simulink model "narrow_FM"  (R2020b)
settings: Solver=VariableStepAuto  StartTime=0.0  StopTime=10.0  RelTol=1e-3
undefined symbols (not defined in the file or in its folder): DiscIntNeverNeededParam
libraries: audiosources x3, dspvision x3, dspfdesign x2, simulink x1
settings Model: Creator=MinsooKang  LastModifiedBy=MinsooKang

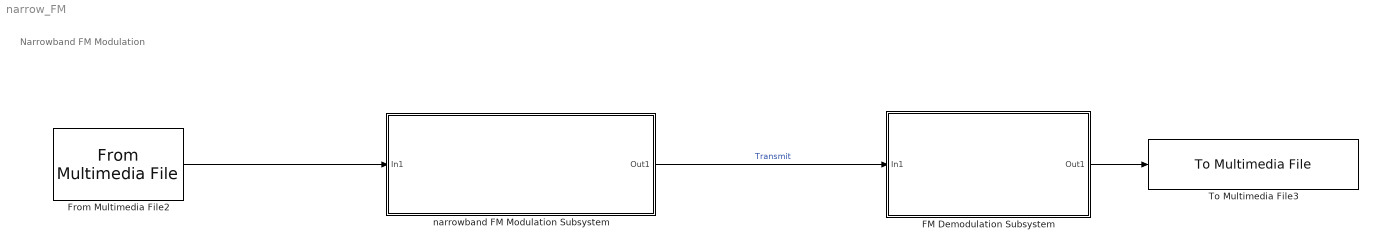
== system narrow_FM ==
  note: Narrowband FM Modulation
  FM Demodulation Subsystem : Subsystem
  From Multimedia File2 : dspvision/From Multimedia File  inputFilename=C:\Users\MinsooKang\Desktop\matlab\audio.flac  readRange=[1 Inf]  loop=on  numPlays=inf  outputStreams=Audio only  videoDataType=single  audioDataType=double  inheritSampleTime=on  userDefinedSampleTime=1/30  noAudioOutput=off  isIntensityVideo=off  fourcc=RGB  colorVideoFormat=Separate color signals  outputEOF=off  dataOrg=Column-major  audioFrameSize=1024  computeAudioFrameSize=off  outSamplingMode=Sample based
  To Multimedia File3 : dspvision/To Multimedia File  outputFilename=C:\Users\MinsooKang\Desktop\matlab\narrow_FM_demodulated.wav  streamSelection=Audio only  videoCompressor=None (uncompressed)  audioCompressor=None (uncompressed)  imagePorts=Separate color signals  fileType=WAV  audioDatatype=32-bit float  fourcc=RGB  videoQuality=75  mj2000CompFactor=10
  narrowband FM Modulation Subsystem : Subsystem
  wires:
  narrowband FM Modulation Subsystem/1(Out1) -> FM Demodulation Subsystem/1(In1)  "Transmit"
  FM Demodulation Subsystem/1(Out1) -> To Multimedia File3/1
  From Multimedia File2/1 -> narrowband FM Modulation Subsystem/1(In1)

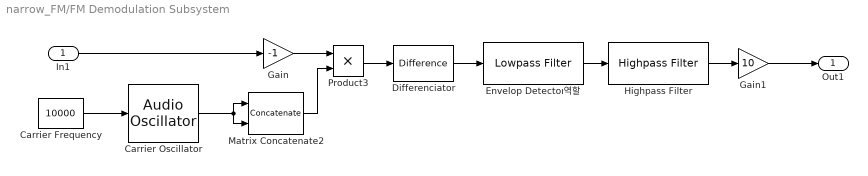
== system narrow_FM/FM Demodulation Subsystem ==
  In1 : Inport
  Carrier Frequency : Constant  Value=10000
  Carrier Oscillator : audiosources/Audio Oscillator  FrequencyPort=on  Frequency=100  AmplitudePort=off  Amplitude=1  DCOffsetPort=off  PhaseOffset=0  DCOffset=0  WidthPort=off  Width=1  DutyCyclePort=off  DutyCycle=0.5  SampsPerFrame=1024  Fs=44100  OutputDataType=double  SimulateUsing=Code generation
      settings: SourceProductBaseCode=AU  SignalType=sine
  Differenciator : simulink/Discrete/Difference  ICPrevInput=0.0  OutMin=[]  OutMax=[]  OutDataType=fixdt(1, 16)  OutScaling=2^-10  DoSatur=off
  Envelop Detector역할 : dspfdesign/Lowpass Filter  FilterType=FIR  DesignForMinimumOrder=on  FilterOrder=50  PassbandFrequency=1500  StopbandFrequency=1600  PassbandRipple=0.1  StopbandAttenuation=80  InheritSampleRate=off  SampleRate=44100  SimulateUsing=Interpreted execution  roundingMode=Floor  coeffsDataTypeStr=fixdt(1,16)
  Gain : Gain  Gain=-1
  Gain1 : Gain  Gain=10
  Highpass Filter : dspfdesign/Highpass Filter  FilterType=FIR  DesignForMinimumOrder=on  FilterOrder=50  StopbandFrequency=20  PassbandFrequency=50  StopbandAttenuation=80  PassbandRipple=0.1  InheritSampleRate=off  SampleRate=44100  SimulateUsing=Interpreted execution  roundingMode=Floor  coeffsDataTypeStr=fixdt(1,16)
  Matrix Concatenate2 : Concatenate  Mode=Multidimensional array  ConcatenateDimension=2
  Product3 : Product
  Out1 : Outport
  wires:
  Differenciator/1 -> Envelop Detector역할/1
  Carrier Frequency/1 -> Carrier Oscillator/1
  Product3/1 -> Differenciator/1
  Carrier Oscillator/1 -> Matrix Concatenate2/2, Matrix Concatenate2/1
  Matrix Concatenate2/1 -> Product3/2
  Envelop Detector역할/1 -> Highpass Filter/1
  Gain/1 -> Product3/1
  In1/1 -> Gain/1
  Highpass Filter/1 -> Gain1/1
  Gain1/1 -> Out1/1

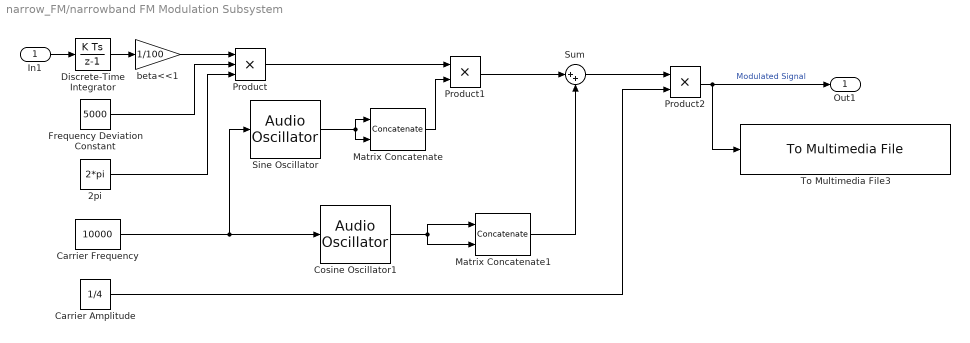
== system narrow_FM/narrowband FM Modulation Subsystem ==
  In1 : Inport
  2pi : Constant  Value=2*pi
  Carrier Amplitude : Constant  Value=1/4
  Carrier Frequency : Constant  Value=10000
  Cosine Oscillator1 : audiosources/Audio Oscillator  FrequencyPort=on  Frequency=100  AmplitudePort=off  Amplitude=1  DCOffsetPort=off  PhaseOffset=0.25  DCOffset=0  WidthPort=off  Width=1  DutyCyclePort=off  DutyCycle=0.5  SampsPerFrame=1024  Fs=44100  OutputDataType=double  SimulateUsing=Code generation
      settings: SourceProductBaseCode=AU  SignalType=sine
  Discrete-Time Integrator : DiscreteIntegrator  SampleTime=-1  ICPrevOutput=DiscIntNeverNeededParam  ICPrevScaledInput=DiscIntNeverNeededParam
  Frequency Deviation Constant : Constant  Value=5000
  Matrix Concatenate : Concatenate  Mode=Multidimensional array  ConcatenateDimension=2
  Matrix Concatenate1 : Concatenate  Mode=Multidimensional array  ConcatenateDimension=2
  Product : Product  Inputs=3
  Product1 : Product
  Product2 : Product
  Sine Oscillator : audiosources/Audio Oscillator  FrequencyPort=on  Frequency=100  AmplitudePort=off  Amplitude=1  DCOffsetPort=off  PhaseOffset=0  DCOffset=0  WidthPort=off  Width=1  DutyCyclePort=off  DutyCycle=0.5  SampsPerFrame=1024  Fs=44100  OutputDataType=double  SimulateUsing=Code generation
      settings: SourceProductBaseCode=AU  SignalType=sine
  Sum : Sum  Inputs=|++
  To Multimedia File3 : dspvision/To Multimedia File  outputFilename=C:\Users\MinsooKang\Desktop\matlab\narrow_FM_modulated.wav  streamSelection=Audio only  videoCompressor=None (uncompressed)  audioCompressor=None (uncompressed)  imagePorts=Separate color signals  fileType=WAV  audioDatatype=32-bit float  fourcc=RGB  videoQuality=75  mj2000CompFactor=10
  beta<<1 : Gain  Gain=1/100
  Out1 : Outport
  wires:
  beta<<1/1 -> Product/1
  Sum/1 -> Product2/1
  Carrier Amplitude/1 -> Product2/2
  Matrix Concatenate1/1 -> Sum/2
  Cosine Oscillator1/1 -> Matrix Concatenate1/2, Matrix Concatenate1/1
  Frequency Deviation Constant/1 -> Product/2
  Product1/1 -> Sum/1
  2pi/1 -> Product/3
  Carrier Frequency/1 -> Sine Oscillator/1, Cosine Oscillator1/1
  Matrix Concatenate/1 -> Product1/2
  Discrete-Time Integrator/1 -> beta<<1/1
  Product/1 -> Product1/1
  Sine Oscillator/1 -> Matrix Concatenate/2, Matrix Concatenate/1
  Product2/1 -> To Multimedia File3/1, Out1/1  "Modulated Signal"
  In1/1 -> Discrete-Time Integrator/1
